simulink model "beautify_model"  (R2018b)
settings: Solver=VariableStepAuto  StartTime=0.0  StopTime=10.0  RelTol=1e-3
values from neighbouring files (symbols this model uses):
  g = 9.81    [state_space_w_kalman_3.m]
  kd_phi = (2*zeta_phi*omega_n_phi-a_phi_1)/a_phi_2    [state_space_w_kalman_3.m]
  ki_chi = omega_chi_phi^2*vg/g    [state_space_w_kalman_3.m]
  kp_chi = 2*zeta_chi*omega_chi_phi*vg/g    [state_space_w_kalman_3.m]
  kp_phi = (aileron_max/error_max)*sign(a_phi_2)    [state_space_w_kalman_3.m]
  roll_rate_noise_power = (0.2*deg2rad)^2    (= 1.21846967915e-05)    [state_space_w_kalman_3.m]
  sensor_fail_time = simtime/2    (= 150)    [state_space_w_kalman_3.m]
  task_nr = 1    [state_space_w_kalman_3.m]
  vg = 580*km_h2m_s    (= 161.111111111)    [state_space_w_kalman_3.m]
  yaw_rate_noise_power = (0.2*deg2rad)^2    (= 1.21846967915e-05)    [state_space_w_kalman_3.m]
libraries: simulink x3, simulink_extras x2
settings Model: Creator=dino  LastModifiedBy=dino

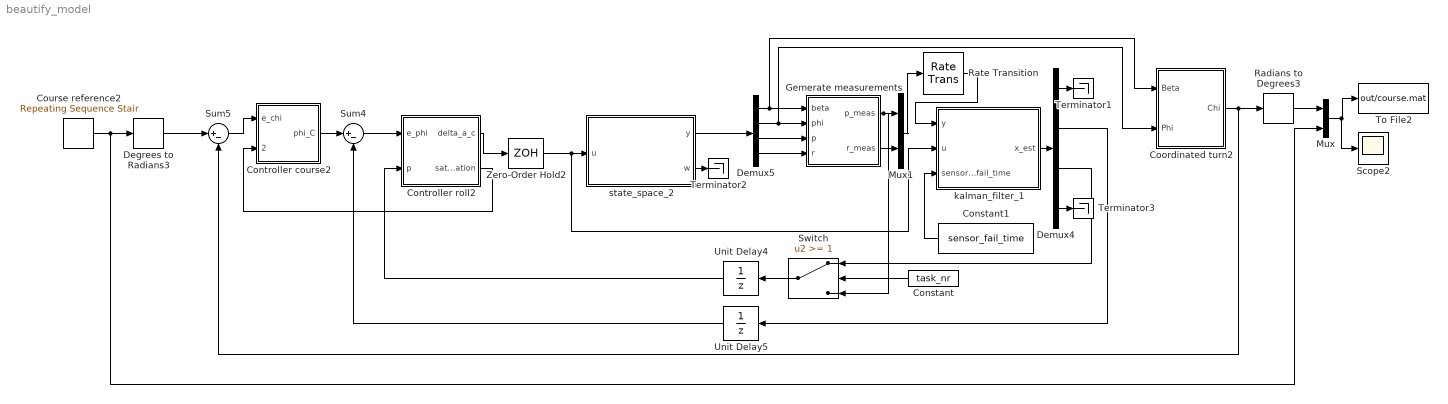
== system beautify_model ==
  Constant : Constant  Value=task_nr
  Constant1 : Constant  Value=sensor_fail_time
  Controller course2 : Subsystem
  Controller roll2 : Subsystem
  Coordinated turn2 : Subsystem
  Course reference2 : simulink/Sources/Repeating Sequence Stair  OutValues=step_series.'  tsamp=60  OutMin=[]  OutMax=[]  OutDataTypeStr=double  OutputDataTypeScalingMode=double  OutDataType=fixdt(0,8)  ConRadixGroup=Best Precision: Vector-wise  OutScaling=2^-12
  Degrees to Radians3 : simulink_extras/Transformations/Degrees to Radians
  Demux4 : Demux
  Demux5 : Demux
  Gemerate measurements : Subsystem
  Mux : Mux  Inputs=2
  Mux1 : Mux  Inputs=2
  Radians to Degrees3 : simulink_extras/Transformations/Radians to Degrees
  Rate Transition : RateTransition  OutPortSampleTime=0.001
  Scope2 : Scope
  Sum4 : Sum  Inputs=|+-
  Sum5 : Sum  Inputs=|+-
  Switch : Switch  Threshold=1
  Terminator1 : Terminator
  Terminator2 : Terminator
  Terminator3 : Terminator
  To File2 : ToFile  Filename=out/course.mat
  Unit Delay4 : UnitDelay  SampleTime=0.01
  Unit Delay5 : UnitDelay  SampleTime=0.01
  Zero-Order Hold2 : ZeroOrderHold  SampleTime=0.01
  kalman_filter_1 : MATLAB Function  TreatAsAtomicUnit=on
  state_space_2 : MATLAB Function  TreatAsAtomicUnit=on
  wires:
  Zero-Order Hold2/1 -> kalman_filter_1/2(u), state_space_2/1(u)
  Mux1/1 -> Rate Transition/1
  Demux4/3 -> Switch/1
  Demux5/4 -> Gemerate measurements/4(r)
  Coordinated turn2/1(Chi) -> Sum5/2, Radians to Degrees3/1
  Mux/1 -> Scope2/1, To File2/1
  Demux5/1 -> Gemerate measurements/1(beta), Coordinated turn2/1(Beta)
  state_space_2/1(y) -> Demux5/1
  Sum4/1 -> Controller roll2/1(e_phi)
  Degrees to Radians3/1 -> Sum5/1
  Constant1/1 -> kalman_filter_1/3(sensor_fail_time)
  kalman_filter_1/1(x_est) -> Demux4/1
  Demux5/2 -> Coordinated turn2/2(Phi), Gemerate measurements/2(phi)
  Gemerate measurements/1(p_meas) -> Switch/3, Mux1/1
  Demux5/3 -> Gemerate measurements/3(p)
  state_space_2/2(w) -> Terminator2/1
  Gemerate measurements/2(r_meas) -> Mux1/2
  Unit Delay4/1 -> Controller roll2/2(p)
  Rate Transition/1 -> kalman_filter_1/1(y)
  Course reference2/1 -> Degrees to Radians3/1, Mux/2
  Controller course2/1(phi_C) -> Sum4/1
  Radians to Degrees3/1 -> Mux/1
  Sum5/1 -> Controller course2/1(e_chi)
  Controller roll2/2(saturation) -> Controller course2/2(saturation)
  Unit Delay5/1 -> Sum4/2
  Controller roll2/1(delta_a_c) -> Zero-Order Hold2/1
  Demux4/2 -> Unit Delay5/1
  Constant/1 -> Switch/2
  Switch/1 -> Unit Delay4/1
  Demux4/1 -> Terminator1/1
  Demux4/4 -> Terminator3/1

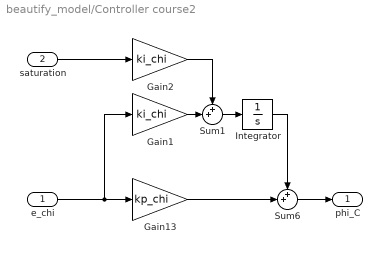
== system beautify_model/Controller course2 ==
  e_chi : Inport
  saturation : Inport  Port=2
  Gain1 : Gain  Gain=ki_chi
  Gain13 : Gain  Gain=kp_chi
  Gain2 : Gain  Gain=ki_chi
  Integrator : Integrator
  Sum1 : Sum  Inputs=++|
  Sum6 : Sum  Inputs=++|
  phi_C : Outport
  wires:
  Gain13/1 -> Sum6/2
  Sum6/1 -> phi_C/1
  e_chi/1 -> Gain1/1, Gain13/1
  Integrator/1 -> Sum6/1
  saturation/1 -> Gain2/1
  Gain1/1 -> Sum1/2
  Sum1/1 -> Integrator/1
  Gain2/1 -> Sum1/1

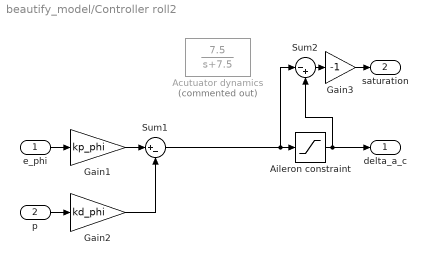
== system beautify_model/Controller roll2 ==
  e_phi : Inport
  p : Inport  Port=2
  Acutuator dynamics : TransferFcn  Commented=on  Numerator=[0 7.5]  Denominator=[1 7.5]
  "Aileron constraint " : Saturate  UpperLimit=30*deg2rad  LowerLimit=-30*deg2rad
  Gain1 : Gain  Gain=kp_phi
  Gain2 : Gain  Gain=kd_phi
  Gain3 : Gain  Gain=-1
  Sum1 : Sum  Inputs=|+-
  Sum2 : Sum  Inputs=|-+
  delta_a_c : Outport
  saturation : Outport  Port=2
  wires:
  Sum1/1 -> Sum2/1, "Aileron constraint "/1
  p/1 -> Gain2/1
  e_phi/1 -> Gain1/1
  "Aileron constraint "/1 -> delta_a_c/1, Sum2/2
  Gain1/1 -> Sum1/1
  Gain2/1 -> Sum1/2
  Sum2/1 -> Gain3/1
  Gain3/1 -> saturation/1

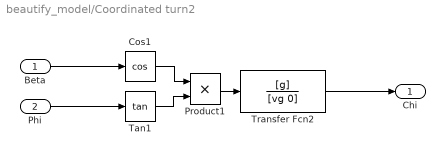
== system beautify_model/Coordinated turn2 ==
  Beta : Inport
  Phi : Inport  Port=2
  Cos1 : Trigonometry  Operator=cos
  Product1 : Product
  Tan1 : Trigonometry  Operator=tan
  Transfer Fcn2 : TransferFcn  Numerator=[g]  Denominator=[vg 0]
  Chi : Outport
  wires:
  Beta/1 -> Cos1/1
  Tan1/1 -> Product1/2
  Cos1/1 -> Product1/1
  Product1/1 -> Transfer Fcn2/1
  Phi/1 -> Tan1/1
  Transfer Fcn2/1 -> Chi/1

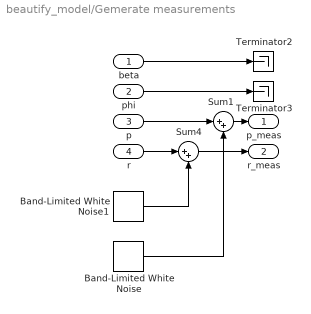
== system beautify_model/Gemerate measurements ==
  beta : Inport
  phi : Inport  Port=2
  p : Inport  Port=3
  r : Inport  Port=4
  Band-Limited White Noise : simulink/Sources/Band-Limited White Noise  Cov=[yaw_rate_noise_power]  Ts=0.01  seed=[23341]
  Band-Limited White Noise1 : simulink/Sources/Band-Limited White Noise  Cov=[roll_rate_noise_power]  Ts=0.01  seed=[53341]
  Sum1 : Sum  Inputs=|++
  Sum4 : Sum  Inputs=|++
  Terminator2 : Terminator
  Terminator3 : Terminator
  p_meas : Outport
  r_meas : Outport  Port=2
  wires:
  beta/1 -> Terminator2/1
  phi/1 -> Terminator3/1
  Sum4/1 -> r_meas/1
  r/1 -> Sum4/1
  Band-Limited White Noise1/1 -> Sum4/2
  Sum1/1 -> p_meas/1
  p/1 -> Sum1/1
  Band-Limited White Noise/1 -> Sum1/2

== matlab function beautify_model/kalman_filter_1 ==
  data: y input; u input; x_est output; sensor_fail_time input
function x_est = kalman_filter_3(y, u, sensor_fail_time)

    % Persistent variables to be kept between function calls
    persistent counter; % Variable for checking if it is the first iteration.
    persistent x_upd;       % The updated state x
    persistent P_upd;       % The updated error covariance
    persistent x_pred;      % The Predicted state x
    persistent P_pred;      % The Predicted error covariance   
    persistent fail_counter; % Variable for checking when to initiate sensor fail
    % Add as well A,B etc. here
    
    h = 0.001;       % Time step (of Euler integration)
    
    if isempty(counter)
        % First iteration
        counter = 1;
        fail_counter = 0;
           
        % Initialize conditions
        x_upd = zeros(4,1); 
        P_upd = eye(4); 
        
    end
    %%%%%%%%%%%%%%%%%%%%%%%%%%%%%%%%%%%%%%%%%%%%%%%%%%%%%%%%%%%%%%%%%%%
    % State-space matrices %%%%%%%%%%%%%%%%%%%%%%%%%%%%%%%%%%%%%%%%%%%%
    %%%%%%%%%%%%%%%%%%%%%%%%%%%%%%%%%%%%%%%%%%%%%%%%%%%%%%%%%%%%%%%%%%%
    A = [-0.322,    0.052,  0.028,  -1.12   ;
         0,         0,      1,      -0.001  ;
         -10.6,     0,      -2.87,  0.46    ;
         6.87,      0,      -0.04,  -0.32   ;];

    B = [0.002; 0; -0.65; -0.02];
    C = [zeros(2), eye(2)];  
    E = eye(4);

    % Discrete version %%%%%%%%%%%%%%%%%%%%%%%%%%%%%%%%%%%%%%%%%%%%%%%%
    Ad = eye(4) + h*A;
    Bd = h*B;  
    Cd = C;
    Ed = E;
    
    %[Ad, Bd] = c2d(A, B, h);  
    
    %%%%%%%%%%%%%%%%%%%%%%%%%%%%%%%%%%%%%%%%%%%%%%%%%%%%%%%%%%%%%%%%%%%
    % Discrete-time Kalman filter algorithm %%%%%%%%%%%%%%%%%%%%%%%%%%%
    %%%%%%%%%%%%%%%%%%%%%%%%%%%%%%%%%%%%%%%%%%%%%%%%%%%%%%%%%%%%%%%%%%%

    % KF coviariance matrices %%%%%%%%%%%%%%%%%%%%%%%%%%%%%%%%%%%%%%%%%
    Q = h*10^-6 * ...
        [0.001  0       0       0   ;
         0      1       0       0   ;
         0      0       100     0   ;
         0      0       0       10  ;];     
    
    fail_counter = fail_counter + 1;
    if (fail_counter * h) >= sensor_fail_time && sensor_fail_time >= 0
        R = 1e20*eye(2);
    else
        R = 10000*(0.2*(pi/180))^2 * ...
            [1      0   ;
             0      1   ;]; 
    end
    % Predict %%%%%%%%%%%%%%%%%%%%%%%%%%%%%%%%%%%%%%%%%%%%%%%%%%%%%%%%%

    % Predicted (a priori) state estimate
    x_pred = Ad * x_upd + Bd * u;        
    % Predicted (a priori) error covariance
    P_pred = Ad * P_upd * Ad' + E * Q * E'; 

    % Update %%%%%%%%%%%%%%%%%%%%%%%%%%%%%%%%%%%%%%%%%%%%%%%%%%%%%%%%%%

    % Innovation or measurement pre-fit residual
    y_tilde = y - C * x_pred;
    % Innovation (or pre-fit residual) covariance
    S = C * P_pred * C' + R;
    % Optimal Kalman gain
    K = P_pred * C' * inv(S);

    % Updated (a posteriori) state estimate
    x_upd = x_pred + K * y_tilde;
    % Updated (a posteriori) estimate covariance
    P_upd = (eye(4) - K * C) * P_pred; 

    % Return output
    x_est = x_upd;  
end

== matlab function beautify_model/state_space_2 ==
  data: u input; y output; w output
function [y, w] = state_space_3(u)
% Generate the output of the state space

    % Persistent variables to be kept between function calls
    persistent counter; % Variable for checking if it is the first iteration.
    persistent x;       % The state x
    
   % The next line is necessary for generating unique process noise for every simulation.
   % Otherwise, the noise will be equal every time you run the simulation,
   % even though it is white. This has to do with how Matlab generates
   % random numbers. 
   coder.extrinsic('randn','rng');
    
    h = 0.01;       % Time step of Euler integration
    delta_a_c = u;  % Aileron input
    
    if isempty(counter)
      % First iteration
        counter = 1;
           
        % Initialize state space
        x = zeros(5,1);
        w = zeros(5,1); 
        rng('shuffle'); % Necessary for generating unique process noise for every simulation.
    
    else
        % State-space matrices
        A = [-0.322, 0.052, 0.028, -1.12, 0.002;
             0, 0, 1, -0.001, 0;
             -10.6, 0, -2.87, 0.46, -0.65;  
             6.87, 0, -0.04, -0.32, -0.02;
             0, 0, 0, 0, -7.5];
 
        B = [0; 0; 0; 0; 7.5;];
        
        E = eye(5);
        
        % Discrete version
        Ad = eye(5) + h*A;
        Bd = h*B;
        Ed = E;
        
        % The Qd matrix in the assignment is given directly in discrete-time here and
        % therefore, it is not necessary to discretize E.
        Qd = h*10^-6*[0.001, 0, 0, 0, 0;
                  0, 1, 0, 0, 0;
                  0, 0, 100, 0, 0;
                  0, 0, 0, 10, 0;
                  0, 0, 0, 0, 0];
          
        w = sqrt(Qd)*randn(5,1,1); % The standard deviation must be multiplied with random numbers with a zero-mean unit variance random number to generate process noise. 
        
        % Discrete-time state space update
        x = Ad*x + Bd * delta_a_c + Ed*w;
    end
    y = x(1:4); % Return every state except the actuator state.
end
